simulink model "rappellingLoop"  (R2013b)
settings: Solver=ode45  StartTime=0.0  StopTime=30  RelTol=1e-12  AbsTol=1e-12
values from neighbouring files (symbols this model uses):
  domain_to_slow = -0.2    [RappellingSimulink.m]    (also in rappelMain.m)
  effective_radius_spool = radius_spool + 3*r_wire    (= 0.04683125)    [RappellingSimulink.m]    (also in rappelMain.m)
  frac_of_domain_to_steps_per_sec = 8000/0.2    (= 40000)    [RappellingSimulink.m]    (also in rappelMain.m)
  radperstep = 2*pi/n_steps_true    (= 0.000261799387799)    [RappellingSimulink.m]    (also in rappelMain.m)
libraries: simulink x1
settings Model: Creator=John Russo  LastModifiedBy=Thomas
settings DataIOCC: FinalStateName=0  InitialState=x0  LimitDataPoints=off  LoadExternalInput=on  LoadInitialState=on  SignalLoggingSaveFormat=ModelDataLogs
settings DebuggingCC: UnderspecifiedInitializationDetection=Simplified  MergeDetectMultiDrivingBlocksExec=error  SolverPrmCheckMsg=none  MultiTaskDSMMsg=warning  MultiTaskCondExecSysMsg=none  InitInArrayFormatMsg=none
settings RTWCC: IncludeERTFirstTime=on
settings GRTTargetCC: CodeReplacementLibrary=None  CPPClassGenCompliant=on

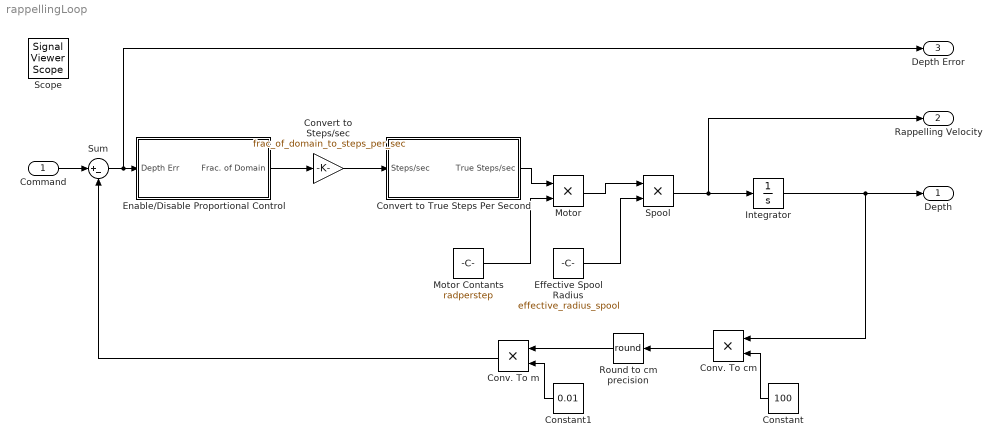
== system rappellingLoop ==
  Command : Inport
  Constant : Constant  Value=100
  Constant1 : Constant  Value=0.01
  Conv. To cm : Product
  Conv. To m : Product
  Convert to Steps/sec : Gain  Gain=frac_of_domain_to_steps_per_sec
  Convert to True Steps Per Second : Subsystem
  Effective Spool Radius : Constant  Value=effective_radius_spool
  Enable/Disable Proportional Control : Subsystem
  Integrator : Integrator
  Motor : Product
  Motor Contants : Constant  Value=radperstep
  Round to cm precision : Rounding  Operator=round
  Spool : Product
  Sum : Sum  Inputs=|+-
  Depth : Outport
  Rappelling Velocity : Outport  Port=2
  Depth Error : Outport  Port=3
  Scope : SignalViewerScope  IOType=viewer  ZoomMode=yonly  RefreshTime=0.035000
      settings: YMin=-10000  YMax=1000
  wires:
  Command/1 -> Sum/1
  Motor Contants/1 -> Motor/2
  Motor/1 -> Spool/1
  Effective Spool Radius/1 -> Spool/2
  Spool/1 -> Rappelling Velocity/1, Integrator/1
  Convert to Steps/sec/1 -> Convert to True Steps Per Second/1(Steps/sec)
  Sum/1 -> Depth Error/1, Enable/Disable Proportional Control/1(Depth Err)
  Conv. To m/1 -> Sum/2
  Conv. To cm/1 -> Round to cm precision/1
  Constant/1 -> Conv. To cm/2
  Round to cm precision/1 -> Conv. To m/1
  Constant1/1 -> Conv. To m/2
  Integrator/1 -> Conv. To cm/1, Depth/1
  Enable/Disable Proportional Control/1(Frac. of Domain) -> Convert to Steps/sec/1
  Convert to True Steps Per Second/1(True Steps/sec) -> Motor/1

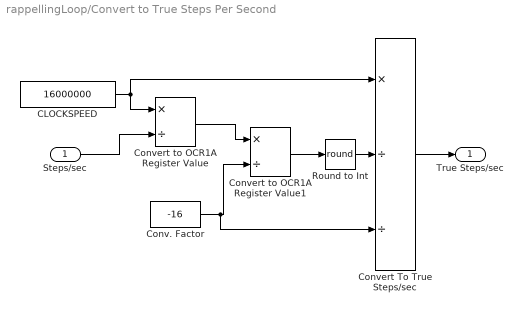
== system rappellingLoop/Convert to True Steps Per Second ==
  Steps/sec : Inport
  CLOCKSPEED : Constant  Value=16000000
  Conv. Factor : Constant  Value=-16
  Convert To True Steps/sec : Product  Inputs=*//
  Convert to OCR1A Register Value : Product  Inputs=*/  RndMeth=Round
  Convert to OCR1A Register Value1 : Product  Inputs=*/  OutMin=124  OutMax=2500  RndMeth=Round
  Round to Int : Rounding  Operator=round
  True Steps/sec : Outport
  wires:
  Steps/sec/1 -> Convert to OCR1A Register Value/2
  Convert to OCR1A Register Value/1 -> Convert to OCR1A Register Value1/1
  Round to Int/1 -> Convert To True Steps/sec/2
  Convert To True Steps/sec/1 -> True Steps/sec/1
  CLOCKSPEED/1 -> Convert to OCR1A Register Value/1, Convert To True Steps/sec/1
  Conv. Factor/1 -> Convert To True Steps/sec/3, Convert to OCR1A Register Value1/2
  Convert to OCR1A Register Value1/1 -> Round to Int/1

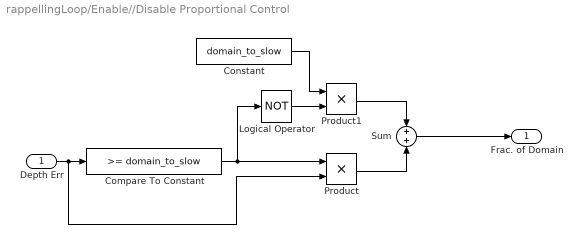
== system rappellingLoop/Enable//Disable Proportional Control ==
  Depth Err : Inport
  Compare To Constant : simulink/Logic and Bit Operations/Compare To Constant  relop=>=  const=domain_to_slow  OutDataTypeStr=uint8
  Constant : Constant  Value=domain_to_slow
  Logical Operator : Logic  Operator=NOT  AllPortsSameDT=off  OutDataTypeStr=boolean
  Product : Product
  Product1 : Product
  Sum : Sum  Inputs=+|+
  Frac. of Domain : Outport
  wires:
  Depth Err/1 -> Product/2, Compare To Constant/1
  Compare To Constant/1 -> Logical Operator/1, Product/1
  Constant/1 -> Product1/1
  Logical Operator/1 -> Product1/2
  Sum/1 -> Frac. of Domain/1
  Product1/1 -> Sum/1
  Product/1 -> Sum/2
